simulink model "B4_quadcopter_model_discrete"  (R2021b)
settings: Solver=VariableStepAuto  StartTime=0.0  StopTime=10  FixedStep=0.002  RelTol=1e-3
values from neighbouring files (symbols this model uses):
  coef_sim_1 = tf_des_d.Denominator{1}(2)    [A11_setup_script_pprz.m]    (also in A1_setup_script.m; A6_slow_actuator.m)
  coef_sim_2 = tf_des_d.Numerator{1}(2)    [A11_setup_script_pprz.m]    (also in A1_setup_script.m; A6_slow_actuator.m)
  doublet_mag = - 0.15    (= -0.15)    [A11_setup_script_pprz.m]    (also in A1_setup_script.m)
  doublet_time = 6    [A11_setup_script_pprz.m]    (also in A1_setup_script.m)
  f_8 = 1    [A11_setup_script_pprz.m]    (also in A1_setup_script.m)
  FILT_CUTOFF = 2*pi*5    (= 31.4159265359)    [A11_setup_script_pprz.m]    (also in A1_setup_script.m)
  FILTER = 1    [A11_setup_script_pprz.m]    (also in A1_setup_script.m)
  G1 = inv(I)*G1_r    [A10_simple_plant.m]    (also in A11_setup_script_pprz.m = G1/scale; A1_setup_script.m = [G1;G1_T])
  G1_simple = inv(I)*G1_r_simple    [A1_setup_script.m]
  G2 = G2/scale    [A11_setup_script_pprz.m]    (also in A1_setup_script.m = (1/sampling_time)*inv(I)*(G2_r))
  h_plate = 0.3    [A11_setup_script_pprz.m]    (also in A1_setup_script.m = 0.16)
  I = eye(3,3)    [A10_simple_plant.m]    (also in A11_setup_script_pprz.m; A1_setup_script.m; A2_B_matrix_generation_symbolic.m = [Ixx 0 0; A3_B_matrix_generation_symbolic_cascaded.m = [Ixx 0 0)
  Iyy = 0.0008    [A11_setup_script_pprz.m]    (also in A1_setup_script.m = 0.0015)
  Izz = 0.000498    [A11_setup_script_pprz.m]    (also in A1_setup_script.m = 0.00015)
  K = 7    [A11_setup_script_pprz.m]    (also in A1_setup_script.m = 10)
  K_act = 50    [A10_simple_plant.m]    (also in A11_setup_script_pprz.m = 20; A1_setup_script.m = 20)
  K_act_outer = diag([K K K_act])    [A1_setup_script.m]
  K_d = 15    [A11_setup_script_pprz.m]    (also in A1_setup_script.m = 25)
  K_dd = K_act    (= 20)    [A11_setup_script_pprz.m]    (also in A1_setup_script.m)
  K_dyn = K    (= 10)    [A1_setup_script.m]
  K_ec = 50    [A11_setup_script_pprz.m]    (also in A1_setup_script.m = 251)
  K_ec_d = 13    [A11_setup_script_pprz.m]    (also in A1_setup_script.m = 25)
  K_ec_d_u = 1.5    [A11_setup_script_pprz.m]    (also in A1_setup_script.m = 5)
  K_ec_d_v = 1.5    [A11_setup_script_pprz.m]    (also in A1_setup_script.m = 5)
  K_ec_d_w = 1.5    [A11_setup_script_pprz.m]    (also in A1_setup_script.m = 5)
  K_ec_dd = 9    [A11_setup_script_pprz.m]    (also in A1_setup_script.m = 45)
  K_ec_i = 0    [A11_setup_script_pprz.m]    (also in A1_setup_script.m = 380)
  K_ec_u = 1.5    [A11_setup_script_pprz.m]    (also in A1_setup_script.m = 5)
  K_ec_v = 1.5    [A11_setup_script_pprz.m]    (also in A1_setup_script.m = 5)
  K_ec_w = 1.5    [A11_setup_script_pprz.m]    (also in A1_setup_script.m = 5)
  K_t = 0.0005    [A10_simple_plant.m]    (also in A11_setup_script_pprz.m = 6.557e-08; A1_setup_script.m = 6.557e-08)
  K_u = 1.0    (= 1)    [A11_setup_script_pprz.m]    (also in A1_setup_script.m = 1.5)
  K_u_d = 2.5    [A11_setup_script_pprz.m]    (also in A1_setup_script.m = 7)
  K_u_dd = K    (= 10)    [A1_setup_script.m]
  K_v = 1.0    (= 1)    [A11_setup_script_pprz.m]    (also in A1_setup_script.m = 1.5)
  K_v_d = 2.5    [A11_setup_script_pprz.m]    (also in A1_setup_script.m = 7)
  K_v_dd = K    (= 10)    [A1_setup_script.m]
  K_w = 1.0    (= 1)    [A11_setup_script_pprz.m]    (also in A1_setup_script.m = 4.5)
  K_w_d = 2.5    [A11_setup_script_pprz.m]    (also in A1_setup_script.m = 7)
  K_w_dd = K    (= 10)    [A1_setup_script.m]
  l_plate = 0.1    [A11_setup_script_pprz.m]    (also in A1_setup_script.m = 0.11)
  m = 0.4    [A10_simple_plant.m]    (also in A11_setup_script_pprz.m; A1_setup_script.m)
  NOISE = 0    [A11_setup_script_pprz.m]    (also in A1_setup_script.m)
  NOISE_ACC = 0.00005    (= 5e-05)    [A11_setup_script_pprz.m]    (also in A1_setup_script.m)
  NOISE_GYRO = 0.00005    (= 5e-05)    [A11_setup_script_pprz.m]    (also in A1_setup_script.m)
  NOISE_RPM = 200    [A11_setup_script_pprz.m]    (also in A1_setup_script.m)
  omega_act = 50    [A6_slow_actuator.m]
  omega_des = 20.00    (= 20)    [A11_setup_script_pprz.m]    (also in A1_setup_script.m; A6_slow_actuator.m = 49)
  sampling_time = 1/frequency    (= 0.002)    [A11_setup_script_pprz.m]    (also in A12_sim_multi_run.m; A1_setup_script.m; A6_slow_actuator.m)
  scale_8 = 1.6    [A11_setup_script_pprz.m]    (also in A1_setup_script.m)
  start_8 = 2    [A11_setup_script_pprz.m]    (also in A1_setup_script.m)
  start_time = 2    [A11_setup_script_pprz.m]    (also in A1_setup_script.m = 1)
  t_8 = 10    [A11_setup_script_pprz.m]    (also in A1_setup_script.m)
  w_plate = 0.3    [A11_setup_script_pprz.m]    (also in A1_setup_script.m = 0.36)
undefined symbols (not defined in the file or in its folder): DiscIntNeverNeededParam, K_ec_d_p, K_ec_d_q, K_ec_d_r, K_ec_dd_p, K_ec_dd_q, K_ec_dd_r, K_ec_i_u, K_ec_i_v, K_ec_i_w, K_ec_p, K_ec_q, K_ec_r, K_p, K_p_d, K_p_dd, K_q, K_q_d, K_q_dd, K_r, K_r_d, K_r_dd
libraries: simulink x44, cstblocks x37, dspinverses x26, dspmathops x9, dspstat3 x9, aerolibutil x9, sharedutil x3, aerolibanim x1
(part 10 of 13)

== system B4_quadcopter_model_discrete/Discrete Model/Discrete INDI Controller Cascaded w// Actuator Compensation1/INTERNAL REFERENCE MODEL ATTITUDE/body rates to euler rates ==
  p : Inport
  q : Inport  Port=2
  r : Inport  Port=3
  Demux : Demux  Outputs=3
  Matrix Multiply : Product  Multiplication=Matrix(*)
  Mux : Mux  Inputs=3
  phi_dot : Outport
  theta_dot : Outport  Port=2
  psi_dot : Outport  Port=3
  wires:
  p/1 -> Mux/1
  q/1 -> Mux/2
  r/1 -> Mux/3
  [T_discr] -> Matrix Multiply/1
  Mux/1 -> Matrix Multiply/2
  Matrix Multiply/1 -> Demux/1
  Demux/3 -> psi_dot/1
  Demux/2 -> theta_dot/1
  Demux/1 -> phi_dot/1

== system B4_quadcopter_model_discrete/Discrete Model/Discrete INDI Controller Cascaded w// Actuator Compensation1/INTERNAL REFERENCE MODEL ATTITUDE/euler rates to body rates ==
  phi_dot : Inport
  theta_dot : Inport  Port=2
  psi_dot : Inport  Port=3
  Demux : Demux  Outputs=3
  Matrix Multiply : Product  Multiplication=Matrix(*)
  Mux : Mux  Inputs=3
  p : Outport
  q : Outport  Port=2
  r : Outport  Port=3
  wires:
  phi_dot/1 -> Mux/1
  theta_dot/1 -> Mux/2
  psi_dot/1 -> Mux/3
  [R_discr] -> Matrix Multiply/1
  Mux/1 -> Matrix Multiply/2
  Matrix Multiply/1 -> Demux/1
  Demux/3 -> r/1
  Demux/2 -> q/1
  Demux/1 -> p/1

== system B4_quadcopter_model_discrete/Discrete Model/Plant and State Estimation/Butterworth Lowpass 2nd Order1/Switch Case Action Subsystem ==
  In1 : Inport
  Action Port : ActionPort  ActionPortLabel=case [ 1 ]:
  Constant5 : Constant  Value=FILT_CUTOFF  SampleTime=sampling_time
  Lowpass2 : cstblocks/Linear Parameter Varying/Discrete Varying Lowpass  N=2  w0=0  Ts=sampling_time
      settings: SourceProductBaseCode=CT
  Out1 : Outport
  wires:
  Constant5/1 -> Lowpass2/2
  In1/1 -> Lowpass2/1
  Lowpass2/1 -> Out1/1

== system B4_quadcopter_model_discrete/Discrete Model/Plant and State Estimation/Butterworth Lowpass 2nd Order1/Switch Case Action Subsystem1 ==
  In1 : Inport
  Action Port : ActionPort  ActionPortLabel=default:
  Out1 : Outport
  wires:
  In1/1 -> Out1/1

== system B4_quadcopter_model_discrete/Discrete Model/Plant and State Estimation/Butterworth Lowpass 2nd Order2/Switch Case Action Subsystem ==
  In1 : Inport
  Action Port : ActionPort  ActionPortLabel=case [ 1 ]:
  Constant5 : Constant  Value=FILT_CUTOFF  SampleTime=sampling_time
  Lowpass2 : cstblocks/Linear Parameter Varying/Discrete Varying Lowpass  N=2  w0=0  Ts=sampling_time
      settings: SourceProductBaseCode=CT
  Out1 : Outport
  wires:
  Constant5/1 -> Lowpass2/2
  In1/1 -> Lowpass2/1
  Lowpass2/1 -> Out1/1

== system B4_quadcopter_model_discrete/Discrete Model/Plant and State Estimation/Butterworth Lowpass 2nd Order2/Switch Case Action Subsystem1 ==
  In1 : Inport
  Action Port : ActionPort  ActionPortLabel=default:
  Out1 : Outport
  wires:
  In1/1 -> Out1/1

== system B4_quadcopter_model_discrete/Discrete Model/Plant and State Estimation/Butterworth Lowpass 2nd Order3/Switch Case Action Subsystem ==
  In1 : Inport
  Action Port : ActionPort  ActionPortLabel=case [ 1 ]:
  Constant5 : Constant  Value=FILT_CUTOFF  SampleTime=sampling_time
  Lowpass2 : cstblocks/Linear Parameter Varying/Discrete Varying Lowpass  N=2  w0=0  Ts=sampling_time
      settings: SourceProductBaseCode=CT
  Out1 : Outport
  wires:
  Constant5/1 -> Lowpass2/2
  In1/1 -> Lowpass2/1
  Lowpass2/1 -> Out1/1

== system B4_quadcopter_model_discrete/Discrete Model/Plant and State Estimation/Butterworth Lowpass 2nd Order3/Switch Case Action Subsystem1 ==
  In1 : Inport
  Action Port : ActionPort  ActionPortLabel=default:
  Out1 : Outport
  wires:
  In1/1 -> Out1/1

== system B4_quadcopter_model_discrete/Discrete Model/Plant and State Estimation/Butterworth Lowpass 2nd Order4/Switch Case Action Subsystem ==
  In1 : Inport
  Action Port : ActionPort  ActionPortLabel=case [ 1 ]:
  Constant5 : Constant  Value=FILT_CUTOFF  SampleTime=sampling_time
  Lowpass2 : cstblocks/Linear Parameter Varying/Discrete Varying Lowpass  N=2  w0=0  Ts=sampling_time
      settings: SourceProductBaseCode=CT
  Out1 : Outport
  wires:
  Constant5/1 -> Lowpass2/2
  In1/1 -> Lowpass2/1
  Lowpass2/1 -> Out1/1

== system B4_quadcopter_model_discrete/Discrete Model/Plant and State Estimation/Butterworth Lowpass 2nd Order4/Switch Case Action Subsystem1 ==
  In1 : Inport
  Action Port : ActionPort  ActionPortLabel=default:
  Out1 : Outport
  wires:
  In1/1 -> Out1/1

== system B4_quadcopter_model_discrete/Discrete Model/Plant and State Estimation/Butterworth Lowpass 2nd Order5/Switch Case Action Subsystem ==
  In1 : Inport
  Action Port : ActionPort  ActionPortLabel=case [ 1 ]:
  Constant5 : Constant  Value=FILT_CUTOFF  SampleTime=sampling_time
  Lowpass2 : cstblocks/Linear Parameter Varying/Discrete Varying Lowpass  N=2  w0=0  Ts=sampling_time
      settings: SourceProductBaseCode=CT
  Out1 : Outport
  wires:
  Constant5/1 -> Lowpass2/2
  In1/1 -> Lowpass2/1
  Lowpass2/1 -> Out1/1

== system B4_quadcopter_model_discrete/Discrete Model/Plant and State Estimation/Butterworth Lowpass 2nd Order5/Switch Case Action Subsystem1 ==
  In1 : Inport
  Action Port : ActionPort  ActionPortLabel=default:
  Out1 : Outport
  wires:
  In1/1 -> Out1/1

== system B4_quadcopter_model_discrete/Discrete Model/Plant and State Estimation/Plant Dynamics Continuous/Disturbance Block ==
  Step : Step  Time=2  After=60  SampleTime=0
  Sum : Sum  Inputs=|++
  Total Disturbance : Outport
  wires:
  Step/1 -> Sum/1
  Sum/1 -> Total Disturbance/1

== system B4_quadcopter_model_discrete/Discrete Model/Plant and State Estimation/Plant Dynamics Continuous/Omega_I_Omega1 ==
  pqr_body : Inport
  Inertia : Inport  Port=2
  3x3 Cross Product : sharedutil/3x3 Cross Product  aMode=aMode
      settings: SourceProductBaseCode=AE,PW,DR,MT,UV,VE
  Matrix Multiply1 : Product  Multiplication=Matrix(*)
  Final product : Outport
  wires:
  Inertia/1 -> Matrix Multiply1/1
  Matrix Multiply1/1 -> 3x3 Cross Product/2
  3x3 Cross Product/1 -> Final product/1
  pqr_body/1 -> 3x3 Cross Product/1, Matrix Multiply1/2

== system B4_quadcopter_model_discrete/Discrete Model - Complementary Filtering/Continuous Actuator Dynamics/Noise RPM/Switch Case Action Subsystem ==
  Action Port : ActionPort  ActionPortLabel=case [ 1 ]:
  RPM Noise : simulink/Sources/Band-Limited White Noise  Cov=[NOISE_RPM]  Ts=sampling_time  seed=[23341]
  Out1 : Outport
  wires:
  RPM Noise/1 -> Out1/1

== system B4_quadcopter_model_discrete/Discrete Model - Complementary Filtering/Continuous Actuator Dynamics/Noise RPM/Switch Case Action Subsystem1 ==
  Action Port : ActionPort  ActionPortLabel=default:
  Constant : Constant  Value=0  SampleTime=sampling_time
  Out1 : Outport
  wires:
  Constant/1 -> Out1/1

== system B4_quadcopter_model_discrete/Discrete Model - Complementary Filtering/Discrete INDI Controller Cascaded/INTERNAL REFERENCE MODEL ATTITUDE/body rates to euler rates ==
  p : Inport
  q : Inport  Port=2
  r : Inport  Port=3
  Demux : Demux  Outputs=3
  Matrix Multiply : Product  Multiplication=Matrix(*)
  Mux : Mux  Inputs=3
  phi_dot : Outport
  theta_dot : Outport  Port=2
  psi_dot : Outport  Port=3
  wires:
  p/1 -> Mux/1
  q/1 -> Mux/2
  r/1 -> Mux/3
  [T_discr] -> Matrix Multiply/1
  Mux/1 -> Matrix Multiply/2
  Matrix Multiply/1 -> Demux/1
  Demux/3 -> psi_dot/1
  Demux/2 -> theta_dot/1
  Demux/1 -> phi_dot/1

== system B4_quadcopter_model_discrete/Discrete Model - Complementary Filtering/Discrete INDI Controller Cascaded/INTERNAL REFERENCE MODEL ATTITUDE/euler rates to body rates ==
  phi_dot : Inport
  theta_dot : Inport  Port=2
  psi_dot : Inport  Port=3
  Demux : Demux  Outputs=3
  Matrix Multiply : Product  Multiplication=Matrix(*)
  Mux : Mux  Inputs=3
  p : Outport
  q : Outport  Port=2
  r : Outport  Port=3
  wires:
  phi_dot/1 -> Mux/1
  theta_dot/1 -> Mux/2
  psi_dot/1 -> Mux/3
  [R_discr] -> Matrix Multiply/1
  Mux/1 -> Matrix Multiply/2
  Matrix Multiply/1 -> Demux/1
  Demux/3 -> r/1
  Demux/2 -> q/1
  Demux/1 -> p/1

== system B4_quadcopter_model_discrete/Discrete Model - Complementary Filtering/Discrete INDI Controller Cascaded/Subsystem1/Doublet Block ==
  Scope : Scope
  Step : Step  Time=start_time  After=doublet_mag  SampleTime=sampling_time
  Step1 : Step  Time=start_time + doublet_time/2  After=-doublet_mag*2  SampleTime=sampling_time
  Step2 : Step  Time=start_time + doublet_time  After=0  SampleTime=sampling_time
  Sum : Sum  Inputs=|++
  Sum1 : Sum  Inputs=|++
  Out1 : Outport
  wires:
  Step/1 -> Sum/1
  Step1/1 -> Sum/2
  Sum/1 -> Sum1/1
  Sum1/1 -> Out1/1, Scope/1
  Step2/1 -> Sum1/2

== system B4_quadcopter_model_discrete/Discrete Model - Complementary Filtering/Discrete INDI Controller Cascaded w// Actuator Compensation/INTERNAL REFERENCE MODEL ATTITUDE/body rates to euler rates ==
  p : Inport
  q : Inport  Port=2
  r : Inport  Port=3
  Demux : Demux  Outputs=3
  Matrix Multiply : Product  Multiplication=Matrix(*)
  Mux : Mux  Inputs=3
  phi_dot : Outport
  theta_dot : Outport  Port=2
  psi_dot : Outport  Port=3
  wires:
  p/1 -> Mux/1
  q/1 -> Mux/2
  r/1 -> Mux/3
  [T_discr] -> Matrix Multiply/1
  Mux/1 -> Matrix Multiply/2
  Matrix Multiply/1 -> Demux/1
  Demux/3 -> psi_dot/1
  Demux/2 -> theta_dot/1
  Demux/1 -> phi_dot/1

== system B4_quadcopter_model_discrete/Discrete Model - Complementary Filtering/Discrete INDI Controller Cascaded w// Actuator Compensation/INTERNAL REFERENCE MODEL ATTITUDE/euler rates to body rates ==
  phi_dot : Inport
  theta_dot : Inport  Port=2
  psi_dot : Inport  Port=3
  Demux : Demux  Outputs=3
  Matrix Multiply : Product  Multiplication=Matrix(*)
  Mux : Mux  Inputs=3
  p : Outport
  q : Outport  Port=2
  r : Outport  Port=3
  wires:
  phi_dot/1 -> Mux/1
  theta_dot/1 -> Mux/2
  psi_dot/1 -> Mux/3
  [R_discr] -> Matrix Multiply/1
  Mux/1 -> Matrix Multiply/2
  Matrix Multiply/1 -> Demux/1
  Demux/3 -> r/1
  Demux/2 -> q/1
  Demux/1 -> p/1

== system B4_quadcopter_model_discrete/Discrete Model - Complementary Filtering/Discrete INDI Controller Cascaded w// Actuator Compensation/Subsystem/body rates to euler rates ==
  p : Inport
  q : Inport  Port=2
  r : Inport  Port=3
  Demux : Demux  Outputs=3
  Matrix Multiply : Product  Multiplication=Matrix(*)
  Mux : Mux  Inputs=3
  phi_dot : Outport
  theta_dot : Outport  Port=2
  psi_dot : Outport  Port=3
  wires:
  p/1 -> Mux/1
  q/1 -> Mux/2
  r/1 -> Mux/3
  [T_discr] -> Matrix Multiply/1
  Mux/1 -> Matrix Multiply/2
  Matrix Multiply/1 -> Demux/1
  Demux/3 -> psi_dot/1
  Demux/2 -> theta_dot/1
  Demux/1 -> phi_dot/1

== system B4_quadcopter_model_discrete/Discrete Model - Complementary Filtering/Discrete INDI Controller Cascaded w// Actuator Compensation/Subsystem/body rates to euler rates1 ==
  p : Inport
  q : Inport  Port=2
  r : Inport  Port=3
  Demux : Demux  Outputs=3
  Matrix Multiply : Product  Multiplication=Matrix(*)
  Mux : Mux  Inputs=3
  phi_dot : Outport
  theta_dot : Outport  Port=2
  psi_dot : Outport  Port=3
  wires:
  p/1 -> Mux/1
  q/1 -> Mux/2
  r/1 -> Mux/3
  [T_discr] -> Matrix Multiply/1
  Mux/1 -> Matrix Multiply/2
  Matrix Multiply/1 -> Demux/1
  Demux/3 -> psi_dot/1
  Demux/2 -> theta_dot/1
  Demux/1 -> phi_dot/1

== system B4_quadcopter_model_discrete/Discrete Model - Complementary Filtering/Discrete INDI Controller Cascaded w// Actuator Compensation/Subsystem/body rates to euler rates2 ==
  p : Inport
  q : Inport  Port=2
  r : Inport  Port=3
  Demux : Demux  Outputs=3
  Matrix Multiply : Product  Multiplication=Matrix(*)
  Mux : Mux  Inputs=3
  phi_dot : Outport
  theta_dot : Outport  Port=2
  psi_dot : Outport  Port=3
  wires:
  p/1 -> Mux/1
  q/1 -> Mux/2
  r/1 -> Mux/3
  [T_discr] -> Matrix Multiply/1
  Mux/1 -> Matrix Multiply/2
  Matrix Multiply/1 -> Demux/1
  Demux/3 -> psi_dot/1
  Demux/2 -> theta_dot/1
  Demux/1 -> phi_dot/1

== system B4_quadcopter_model_discrete/Discrete Model - Complementary Filtering/Discrete INDI Controller Cascaded w// Actuator Compensation Double/Butterworth Lowpass 2nd Order3/Switch Case Action Subsystem ==
  In1 : Inport
  Action Port : ActionPort
  Constant5 : Constant  Value=FILT_CUTOFF  SampleTime=sampling_time
  Lowpass2 : cstblocks/Linear Parameter Varying/Discrete Varying Lowpass  N=2  w0=0  Ts=sampling_time
      settings: SourceProductBaseCode=CT
  Out1 : Outport
  wires:
  Constant5/1 -> Lowpass2/2
  In1/1 -> Lowpass2/1
  Lowpass2/1 -> Out1/1

== system B4_quadcopter_model_discrete/Discrete Model - Complementary Filtering/Discrete INDI Controller Cascaded w// Actuator Compensation Double/Butterworth Lowpass 2nd Order3/Switch Case Action Subsystem1 ==
  In1 : Inport
  Action Port : ActionPort
  Out1 : Outport
  wires:
  In1/1 -> Out1/1

== system B4_quadcopter_model_discrete/Discrete Model - Complementary Filtering/Discrete INDI Controller Cascaded w// Actuator Compensation Double/INTERNAL REFERENCE MODEL ATTITUDE/body rates to euler rates ==
  p : Inport
  q : Inport  Port=2
  r : Inport  Port=3
  Demux : Demux  Outputs=3
  Matrix Multiply : Product  Multiplication=Matrix(*)
  Mux : Mux  Inputs=3
  phi_dot : Outport
  theta_dot : Outport  Port=2
  psi_dot : Outport  Port=3
  wires:
  p/1 -> Mux/1
  q/1 -> Mux/2
  r/1 -> Mux/3
  [T_discr] -> Matrix Multiply/1
  Mux/1 -> Matrix Multiply/2
  Matrix Multiply/1 -> Demux/1
  Demux/3 -> psi_dot/1
  Demux/2 -> theta_dot/1
  Demux/1 -> phi_dot/1

== system B4_quadcopter_model_discrete/Discrete Model - Complementary Filtering/Discrete INDI Controller Cascaded w// Actuator Compensation Double/INTERNAL REFERENCE MODEL ATTITUDE/euler rates to body rates ==
  phi_dot : Inport
  theta_dot : Inport  Port=2
  psi_dot : Inport  Port=3
  Demux : Demux  Outputs=3
  Matrix Multiply : Product  Multiplication=Matrix(*)
  Mux : Mux  Inputs=3
  p : Outport
  q : Outport  Port=2
  r : Outport  Port=3
  wires:
  phi_dot/1 -> Mux/1
  theta_dot/1 -> Mux/2
  psi_dot/1 -> Mux/3
  [R_discr] -> Matrix Multiply/1
  Mux/1 -> Matrix Multiply/2
  Matrix Multiply/1 -> Demux/1
  Demux/3 -> r/1
  Demux/2 -> q/1
  Demux/1 -> p/1

== system B4_quadcopter_model_discrete/Discrete Model - Complementary Filtering/Discrete INDI Controller Cascaded w// Actuator Compensation Double/Pitch Jerk Compensation/Butterworth Lowpass 2nd Order2 ==
  state estimate : Inport
  Constant5 : Constant  Value=FILT_CUTOFF  SampleTime=sampling_time
  Lowpass2 : cstblocks/Linear Parameter Varying/Discrete Varying Lowpass  N=2  w0=0  Ts=sampling_time
      settings: SourceProductBaseCode=CT
  Out : Outport
  wires:
  Constant5/1 -> Lowpass2/2
  Lowpass2/1 -> Out/1
  state estimate/1 -> Lowpass2/1

== system B4_quadcopter_model_discrete/Discrete Model - Complementary Filtering/Discrete INDI Controller Cascaded w// Actuator Compensation Double/Pitch Jerk Compensation/Model Based State Estimate ==
  Mux : Mux  Inputs=12
  state estimate : Outport
  wires:
  [Az] -> Mux/9
  [Vy] -> Mux/2
  [q] -> Mux/11
  [phi] -> Mux/4
  [Ay] -> Mux/8
  [p] -> Mux/10
  [psi] -> Mux/6
  [Ax] -> Mux/7
  [r] -> Mux/12
  [Vx] -> Mux/1
  [theta] -> Mux/5
  [Vz] -> Mux/3
  Mux/1 -> state estimate/1  "plant based"

== system B4_quadcopter_model_discrete/Discrete Model - Complementary Filtering/Discrete INDI Controller Cascaded w// Actuator Compensation Double/Pitch Jerk Compensation/State Filtered ==
  Mux : Mux  Inputs=12
  state filtered : Outport
  wires:
  [Az_f] -> Mux/9
  [Vy_f] -> Mux/2
  [q_f] -> Mux/11
  [phi_f] -> Mux/4
  [Ay_f] -> Mux/8
  [p_f] -> Mux/10
  [psi_f] -> Mux/6
  [Ax_f] -> Mux/7
  [r_f] -> Mux/12
  [Vx_f] -> Mux/1
  [theta_f] -> Mux/5
  [Vz_f] -> Mux/3
  Mux/1 -> state filtered/1  "plant based"

== system B4_quadcopter_model_discrete/Discrete Model - Complementary Filtering/Discrete INDI Controller Cascaded w// Actuator Compensation Double/Pitch Jerk Compensation CopyPaste/Aero Package Easy ==
  Constant : Constant  Value=0
  Constant2 : Constant  Value=w_plate
  Constant3 : Constant  Value=h_plate
  Constant5 : Constant  Value=l_plate
  Mux : Mux  Inputs=3
  Mux1 : Mux  Inputs=3
  Terminator : Terminator
  Terminator1 : Terminator
  drag plate My : MATLAB Function  TreatAsAtomicUnit=on
  Aero Moment : Outport
  Aero Force : Outport  Port=2
  wires:
  Mux/1 -> Aero Moment/1  "aero_moment"
  Constant/1 -> Mux1/2, Mux/3, Mux/1
  drag plate My/1(My_dp) -> Mux/2  "My_dp"
  drag plate My/2(Fx_earth) -> Mux1/1  "Fx_aero_earth"
  Constant2/1 -> drag plate My/1(w_plate)
  Constant3/1 -> drag plate My/2(h_plate)
  Constant5/1 -> drag plate My/3(l_plate)
  [theta_cont] -> drag plate My/4(theta)
  Mux1/1 -> Aero Force/1  "aero_force"
  drag plate My/3(Fz_earth) -> Mux1/3  "Fz_aero_earth"
  drag plate My/4(Cl) -> Terminator/1  "Cl"
  drag plate My/5(Cd) -> Terminator1/1  "Cd"
  [u_cont] -> drag plate My/5(u)
  [w_cont] -> drag plate My/6(w)

== system B4_quadcopter_model_discrete/Discrete Model - Complementary Filtering/Discrete INDI Controller Cascaded w// Actuator Compensation Double/Pitch Jerk Compensation1/body rates to euler rates ==
  p : Inport
  q : Inport  Port=2
  r : Inport  Port=3
  Demux : Demux  Outputs=3
  Matrix Multiply : Product  Multiplication=Matrix(*)
  Mux : Mux  Inputs=3
  phi_dot : Outport
  theta_dot : Outport  Port=2
  psi_dot : Outport  Port=3
  wires:
  p/1 -> Mux/1
  q/1 -> Mux/2
  r/1 -> Mux/3
  [T_discr] -> Matrix Multiply/1
  Mux/1 -> Matrix Multiply/2
  Matrix Multiply/1 -> Demux/1
  Demux/3 -> psi_dot/1
  Demux/2 -> theta_dot/1
  Demux/1 -> phi_dot/1

== system B4_quadcopter_model_discrete/Discrete Model - Complementary Filtering/Plant and State Estimation/Angular Velocity Model/Drag Plate Aerodynamics ==
  Constant : Constant  Value=0
  Constant2 : Constant  Value=w_plate
  Constant3 : Constant  Value=h_plate
  Constant5 : Constant  Value=l_plate
  Mux : Mux  Inputs=3
  Mux1 : Mux  Inputs=3
  Scope : Scope  NumInputPorts=2
  drag plate My : MATLAB Function  TreatAsAtomicUnit=on
  Aero Moment : Outport
  Aero Force : Outport  Port=2
  wires:
  drag plate My/2(Fx_earth) -> Mux1/1  "Fx_aero_earth"
  Constant/1 -> Mux/2, Mux/1
  [Vx_cont] -> drag plate My/5(Vx)
  drag plate My/3(Fy_earth) -> Mux1/2  "Fy_aero_earth"
  Constant5/1 -> drag plate My/3(l_plate)
  Mux1/1 -> Aero Force/1  "aero_force"
  [theta_cont] -> drag plate My/4(theta)
  [q_cont] -> drag plate My/8(q)
  drag plate My/5(D_plate_vel) -> Scope/1
  [Vy_cont] -> drag plate My/6(Vy)
  drag plate My/4(Fz_earth) -> Mux1/3  "Fz_aero_earth"
  [psi_cont] -> drag plate My/7(heading)
  Mux/1 -> Aero Moment/1  "aero_moment"
  Constant2/1 -> drag plate My/1(w_plate)
  Constant3/1 -> drag plate My/2(h_plate)
  drag plate My/6(D_plate_rot) -> Scope/2
  drag plate My/1(Mz_dp) -> Mux/3  "Mz_dp"

== system B4_quadcopter_model_discrete/Discrete Model - Complementary Filtering/Plant and State Estimation/Complementary Filter/Butterworth Lowpass 2nd Order1 ==
  In : Inport
  Constant : Constant  Value=FILTER  SampleTime=sampling_time
  Merge : Merge
  Switch Case : SwitchCase
  Switch Case Action Subsystem : Subsystem  TreatAsAtomicUnit=on
  Switch Case Action Subsystem1 : Subsystem  TreatAsAtomicUnit=on
  Out : Outport
  wires:
  Merge/1 -> Out/1
  Switch Case Action Subsystem/1(Out1) -> Merge/1
  Constant/1 -> Switch Case/1
  Switch Case Action Subsystem1/1(Out1) -> Merge/2
  Switch Case/2 -> Switch Case Action Subsystem1/Action
  In/1 -> Switch Case Action Subsystem/1(In1), Switch Case Action Subsystem1/1(In1)
  Switch Case/1 -> Switch Case Action Subsystem/Action

== system B4_quadcopter_model_discrete/Discrete Model - Complementary Filtering/Plant and State Estimation/Complementary Filter/Butterworth Lowpass 2nd Order2 ==
  In : Inport
  Constant : Constant  Value=FILTER  SampleTime=sampling_time
  Merge : Merge
  Switch Case : SwitchCase
  Switch Case Action Subsystem : Subsystem  TreatAsAtomicUnit=on
  Switch Case Action Subsystem1 : Subsystem  TreatAsAtomicUnit=on
  Out : Outport
  wires:
  Merge/1 -> Out/1
  Switch Case Action Subsystem/1(Out1) -> Merge/1
  Constant/1 -> Switch Case/1
  Switch Case Action Subsystem1/1(Out1) -> Merge/2
  Switch Case/2 -> Switch Case Action Subsystem1/Action
  In/1 -> Switch Case Action Subsystem/1(In1), Switch Case Action Subsystem1/1(In1)
  Switch Case/1 -> Switch Case Action Subsystem/Action

== system B4_quadcopter_model_discrete/Discrete Model - Complementary Filtering/Plant and State Estimation/Complementary Filter1/Butterworth Lowpass 2nd Order1 ==
  In : Inport
  Constant : Constant  Value=FILTER  SampleTime=sampling_time
  Merge : Merge
  Switch Case : SwitchCase
  Switch Case Action Subsystem : Subsystem  TreatAsAtomicUnit=on
  Switch Case Action Subsystem1 : Subsystem  TreatAsAtomicUnit=on
  Out : Outport
  wires:
  Merge/1 -> Out/1
  Switch Case Action Subsystem/1(Out1) -> Merge/1
  Constant/1 -> Switch Case/1
  Switch Case Action Subsystem1/1(Out1) -> Merge/2
  Switch Case/2 -> Switch Case Action Subsystem1/Action
  In/1 -> Switch Case Action Subsystem/1(In1), Switch Case Action Subsystem1/1(In1)
  Switch Case/1 -> Switch Case Action Subsystem/Action

== system B4_quadcopter_model_discrete/Discrete Model - Complementary Filtering/Plant and State Estimation/Complementary Filter1/Butterworth Lowpass 2nd Order2 ==
  In : Inport
  Constant : Constant  Value=FILTER  SampleTime=sampling_time
  Merge : Merge
  Switch Case : SwitchCase
  Switch Case Action Subsystem : Subsystem  TreatAsAtomicUnit=on
  Switch Case Action Subsystem1 : Subsystem  TreatAsAtomicUnit=on
  Out : Outport
  wires:
  Merge/1 -> Out/1
  Switch Case Action Subsystem/1(Out1) -> Merge/1
  Constant/1 -> Switch Case/1
  Switch Case Action Subsystem1/1(Out1) -> Merge/2
  Switch Case/2 -> Switch Case Action Subsystem1/Action
  In/1 -> Switch Case Action Subsystem/1(In1), Switch Case Action Subsystem1/1(In1)
  Switch Case/1 -> Switch Case Action Subsystem/Action

== system B4_quadcopter_model_discrete/Discrete Model - Complementary Filtering/Plant and State Estimation/Noise Acc/Switch Case Action Subsystem ==
  Action Port : ActionPort  ActionPortLabel=case [ 1 ]:
  Acc Noise : simulink/Sources/Band-Limited White Noise  Cov=[NOISE_ACC]  Ts=sampling_time  seed=[23341]
  Out1 : Outport
  wires:
  Acc Noise/1 -> Out1/1

== system B4_quadcopter_model_discrete/Discrete Model - Complementary Filtering/Plant and State Estimation/Noise Acc/Switch Case Action Subsystem1 ==
  Action Port : ActionPort  ActionPortLabel=default:
  Constant : Constant  Value=0  SampleTime=sampling_time
  Out1 : Outport
  wires:
  Constant/1 -> Out1/1

== system B4_quadcopter_model_discrete/Discrete Model - Complementary Filtering/Plant and State Estimation/Noise Gyro/Switch Case Action Subsystem ==
  Action Port : ActionPort  ActionPortLabel=case [ 1 ]:
  Gyro Noise : simulink/Sources/Band-Limited White Noise  Cov=[NOISE_GYRO]  Ts=sampling_time  seed=[23341]
  Out1 : Outport
  wires:
  Gyro Noise/1 -> Out1/1

== system B4_quadcopter_model_discrete/Discrete Model - Complementary Filtering/Plant and State Estimation/Noise Gyro/Switch Case Action Subsystem1 ==
  Action Port : ActionPort  ActionPortLabel=default:
  Constant : Constant  Value=0  SampleTime=sampling_time
  Out1 : Outport
  wires:
  Constant/1 -> Out1/1

== system B4_quadcopter_model_discrete/Discrete Model - Complementary Filtering/Plant and State Estimation/Plant Dynamics Continuous/Disturbance Block ==
  Step : Step  Time=2  After=60  SampleTime=0
  Sum : Sum  Inputs=|++
  Total Disturbance : Outport
  wires:
  Step/1 -> Sum/1
  Sum/1 -> Total Disturbance/1

== system B4_quadcopter_model_discrete/Discrete Model - Complementary Filtering/Plant and State Estimation/Plant Dynamics Continuous/Omega_I_Omega1 ==
  pqr_body : Inport
  Inertia : Inport  Port=2
  3x3 Cross Product : sharedutil/3x3 Cross Product  aMode=aMode
      settings: SourceProductBaseCode=AE,PW,DR,MT,UV,VE
  Matrix Multiply1 : Product  Multiplication=Matrix(*)
  Final product : Outport
  wires:
  Inertia/1 -> Matrix Multiply1/1
  Matrix Multiply1/1 -> 3x3 Cross Product/2
  3x3 Cross Product/1 -> Final product/1
  pqr_body/1 -> 3x3 Cross Product/1, Matrix Multiply1/2

== system B4_quadcopter_model_discrete/Discrete Model - Doublet/Continuous Actuator Dynamics/Butterworth Lowpass 2nd Order1/Switch Case Action Subsystem ==
  In1 : Inport
  Action Port : ActionPort  ActionPortLabel=case [ 1 ]:
  Constant5 : Constant  Value=FILT_CUTOFF  SampleTime=sampling_time
  Lowpass2 : cstblocks/Linear Parameter Varying/Discrete Varying Lowpass  N=2  w0=0  Ts=sampling_time
      settings: SourceProductBaseCode=CT
  Out1 : Outport
  wires:
  Constant5/1 -> Lowpass2/2
  In1/1 -> Lowpass2/1
  Lowpass2/1 -> Out1/1

== system B4_quadcopter_model_discrete/Discrete Model - Doublet/Continuous Actuator Dynamics/Butterworth Lowpass 2nd Order1/Switch Case Action Subsystem1 ==
  In1 : Inport
  Action Port : ActionPort  ActionPortLabel=default:
  Out1 : Outport
  wires:
  In1/1 -> Out1/1

== system B4_quadcopter_model_discrete/Discrete Model - Doublet/Discrete INDI Controller Cascaded/INTERNAL REFERENCE MODEL ATTITUDE/body rates to euler rates ==
  p : Inport
  q : Inport  Port=2
  r : Inport  Port=3
  Demux : Demux  Outputs=3
  Matrix Multiply : Product  Multiplication=Matrix(*)
  Mux : Mux  Inputs=3
  phi_dot : Outport
  theta_dot : Outport  Port=2
  psi_dot : Outport  Port=3
  wires:
  p/1 -> Mux/1
  q/1 -> Mux/2
  r/1 -> Mux/3
  [T_discr] -> Matrix Multiply/1
  Mux/1 -> Matrix Multiply/2
  Matrix Multiply/1 -> Demux/1
  Demux/3 -> psi_dot/1
  Demux/2 -> theta_dot/1
  Demux/1 -> phi_dot/1

== system B4_quadcopter_model_discrete/Discrete Model - Doublet/Discrete INDI Controller Cascaded/INTERNAL REFERENCE MODEL ATTITUDE/euler rates to body rates ==
  phi_dot : Inport
  theta_dot : Inport  Port=2
  psi_dot : Inport  Port=3
  Demux : Demux  Outputs=3
  Matrix Multiply : Product  Multiplication=Matrix(*)
  Mux : Mux  Inputs=3
  p : Outport
  q : Outport  Port=2
  r : Outport  Port=3
  wires:
  phi_dot/1 -> Mux/1
  theta_dot/1 -> Mux/2
  psi_dot/1 -> Mux/3
  [R_discr] -> Matrix Multiply/1
  Mux/1 -> Matrix Multiply/2
  Matrix Multiply/1 -> Demux/1
  Demux/3 -> r/1
  Demux/2 -> q/1
  Demux/1 -> p/1

== system B4_quadcopter_model_discrete/Discrete Model - Doublet/Discrete INDI Controller Cascaded/Subsystem/Doublet Block ==
  Scope : Scope
  Step : Step  Time=start_time  After=doublet_mag  SampleTime=sampling_time
  Step1 : Step  Time=start_time + doublet_time/2  After=-doublet_mag*2  SampleTime=sampling_time
  Step2 : Step  Time=start_time + doublet_time  After=0  SampleTime=sampling_time
  Sum : Sum  Inputs=|++
  Sum1 : Sum  Inputs=|++
  Out1 : Outport
  wires:
  Step/1 -> Sum/1
  Step1/1 -> Sum/2
  Sum/1 -> Sum1/1
  Sum1/1 -> Out1/1, Scope/1
  Step2/1 -> Sum1/2

== system B4_quadcopter_model_discrete/Discrete Model - Doublet/Discrete INDI Controller Cascaded w// Actuator Compensation/INTERNAL REFERENCE MODEL ATTITUDE/body rates to euler rates ==
  p : Inport
  q : Inport  Port=2
  r : Inport  Port=3
  Demux : Demux  Outputs=3
  Matrix Multiply : Product  Multiplication=Matrix(*)
  Mux : Mux  Inputs=3
  phi_dot : Outport
  theta_dot : Outport  Port=2
  psi_dot : Outport  Port=3
  wires:
  p/1 -> Mux/1
  q/1 -> Mux/2
  r/1 -> Mux/3
  [T_discr] -> Matrix Multiply/1
  Mux/1 -> Matrix Multiply/2
  Matrix Multiply/1 -> Demux/1
  Demux/3 -> psi_dot/1
  Demux/2 -> theta_dot/1
  Demux/1 -> phi_dot/1

== system B4_quadcopter_model_discrete/Discrete Model - Doublet/Discrete INDI Controller Cascaded w// Actuator Compensation/INTERNAL REFERENCE MODEL ATTITUDE/euler rates to body rates ==
  phi_dot : Inport
  theta_dot : Inport  Port=2
  psi_dot : Inport  Port=3
  Demux : Demux  Outputs=3
  Matrix Multiply : Product  Multiplication=Matrix(*)
  Mux : Mux  Inputs=3
  p : Outport
  q : Outport  Port=2
  r : Outport  Port=3
  wires:
  phi_dot/1 -> Mux/1
  theta_dot/1 -> Mux/2
  psi_dot/1 -> Mux/3
  [R_discr] -> Matrix Multiply/1
  Mux/1 -> Matrix Multiply/2
  Matrix Multiply/1 -> Demux/1
  Demux/3 -> r/1
  Demux/2 -> q/1
  Demux/1 -> p/1

== system B4_quadcopter_model_discrete/Discrete Model - Doublet/Discrete INDI Controller Cascaded w// Actuator Compensation/Subsystem/Doublet Block ==
  Scope : Scope
  Step : Step  Time=start_time  After=doublet_mag  SampleTime=sampling_time
  Step1 : Step  Time=start_time + doublet_time/2  After=-doublet_mag*2  SampleTime=sampling_time
  Step2 : Step  Time=start_time + doublet_time  After=0  SampleTime=sampling_time
  Sum : Sum  Inputs=|++
  Sum1 : Sum  Inputs=|++
  Out1 : Outport
  wires:
  Step/1 -> Sum/1
  Step1/1 -> Sum/2
  Sum/1 -> Sum1/1
  Sum1/1 -> Out1/1, Scope/1
  Step2/1 -> Sum1/2

== system B4_quadcopter_model_discrete/Discrete Model - Doublet/Discrete INDI Controller Cascaded w// Actuator Compensation Double/Butterworth Lowpass 2nd Order3/Switch Case Action Subsystem ==
  In1 : Inport
  Action Port : ActionPort
  Constant5 : Constant  Value=FILT_CUTOFF  SampleTime=sampling_time
  Lowpass2 : cstblocks/Linear Parameter Varying/Discrete Varying Lowpass  N=2  w0=0  Ts=sampling_time
      settings: SourceProductBaseCode=CT
  Out1 : Outport
  wires:
  Constant5/1 -> Lowpass2/2
  In1/1 -> Lowpass2/1
  Lowpass2/1 -> Out1/1

== system B4_quadcopter_model_discrete/Discrete Model - Doublet/Discrete INDI Controller Cascaded w// Actuator Compensation Double/Butterworth Lowpass 2nd Order3/Switch Case Action Subsystem1 ==
  In1 : Inport
  Action Port : ActionPort
  Out1 : Outport
  wires:
  In1/1 -> Out1/1

== system B4_quadcopter_model_discrete/Discrete Model - Doublet/Discrete INDI Controller Cascaded w// Actuator Compensation Double/INTERNAL REFERENCE MODEL ATTITUDE/body rates to euler rates ==
  p : Inport
  q : Inport  Port=2
  r : Inport  Port=3
  Demux : Demux  Outputs=3
  Matrix Multiply : Product  Multiplication=Matrix(*)
  Mux : Mux  Inputs=3
  phi_dot : Outport
  theta_dot : Outport  Port=2
  psi_dot : Outport  Port=3
  wires:
  p/1 -> Mux/1
  q/1 -> Mux/2
  r/1 -> Mux/3
  [T_discr] -> Matrix Multiply/1
  Mux/1 -> Matrix Multiply/2
  Matrix Multiply/1 -> Demux/1
  Demux/3 -> psi_dot/1
  Demux/2 -> theta_dot/1
  Demux/1 -> phi_dot/1

== system B4_quadcopter_model_discrete/Discrete Model - Doublet/Discrete INDI Controller Cascaded w// Actuator Compensation Double/INTERNAL REFERENCE MODEL ATTITUDE/euler rates to body rates ==
  phi_dot : Inport
  theta_dot : Inport  Port=2
  psi_dot : Inport  Port=3
  Demux : Demux  Outputs=3
  Matrix Multiply : Product  Multiplication=Matrix(*)
  Mux : Mux  Inputs=3
  p : Outport
  q : Outport  Port=2
  r : Outport  Port=3
  wires:
  phi_dot/1 -> Mux/1
  theta_dot/1 -> Mux/2
  psi_dot/1 -> Mux/3
  [R_discr] -> Matrix Multiply/1
  Mux/1 -> Matrix Multiply/2
  Matrix Multiply/1 -> Demux/1
  Demux/3 -> r/1
  Demux/2 -> q/1
  Demux/1 -> p/1

== system B4_quadcopter_model_discrete/Discrete Model - Doublet/Discrete INDI Controller Cascaded w// Actuator Compensation Double/Pitch Jerk Compensation/Butterworth Lowpass 2nd Order2 ==
  state estimate : Inport
  Constant5 : Constant  Value=FILT_CUTOFF  SampleTime=sampling_time
  Lowpass2 : cstblocks/Linear Parameter Varying/Discrete Varying Lowpass  N=2  w0=0  Ts=sampling_time
      settings: SourceProductBaseCode=CT
  Out : Outport
  wires:
  Constant5/1 -> Lowpass2/2
  Lowpass2/1 -> Out/1
  state estimate/1 -> Lowpass2/1

== system B4_quadcopter_model_discrete/Discrete Model - Doublet/Discrete INDI Controller Cascaded w// Actuator Compensation Double/Pitch Jerk Compensation/Model Based State Estimate ==
  Mux : Mux  Inputs=12
  state estimate : Outport
  wires:
  [Az] -> Mux/9
  [Vy] -> Mux/2
  [q] -> Mux/11
  [phi] -> Mux/4
  [Ay] -> Mux/8
  [p] -> Mux/10
  [psi] -> Mux/6
  [Ax] -> Mux/7
  [r] -> Mux/12
  [Vx] -> Mux/1
  [theta] -> Mux/5
  [Vz] -> Mux/3
  Mux/1 -> state estimate/1  "plant based"

== system B4_quadcopter_model_discrete/Discrete Model - Doublet/Discrete INDI Controller Cascaded w// Actuator Compensation Double/Pitch Jerk Compensation/State Filtered ==
  Mux : Mux  Inputs=12
  state filtered : Outport
  wires:
  [Az_f] -> Mux/9
  [Vy_f] -> Mux/2
  [q_f] -> Mux/11
  [phi_f] -> Mux/4
  [Ay_f] -> Mux/8
  [p_f] -> Mux/10
  [psi_f] -> Mux/6
  [Ax_f] -> Mux/7
  [r_f] -> Mux/12
  [Vx_f] -> Mux/1
  [theta_f] -> Mux/5
  [Vz_f] -> Mux/3
  Mux/1 -> state filtered/1  "plant based"

== system B4_quadcopter_model_discrete/Discrete Model - Doublet/Discrete INDI Controller Cascaded w// Actuator Compensation Double/Pitch Jerk Compensation CopyPaste/Aero Package Easy ==
  Constant : Constant  Value=0
  Constant2 : Constant  Value=w_plate
  Constant3 : Constant  Value=h_plate
  Constant5 : Constant  Value=l_plate
  Mux : Mux  Inputs=3
  Mux1 : Mux  Inputs=3
  Terminator : Terminator
  Terminator1 : Terminator
  drag plate My : MATLAB Function  TreatAsAtomicUnit=on
  Aero Moment : Outport
  Aero Force : Outport  Port=2
  wires:
  Mux/1 -> Aero Moment/1  "aero_moment"
  Constant/1 -> Mux1/2, Mux/3, Mux/1
  drag plate My/1(My_dp) -> Mux/2  "My_dp"
  drag plate My/2(Fx_earth) -> Mux1/1  "Fx_aero_earth"
  Constant2/1 -> drag plate My/1(w_plate)
  Constant3/1 -> drag plate My/2(h_plate)
  Constant5/1 -> drag plate My/3(l_plate)
  [theta_cont] -> drag plate My/4(theta)
  Mux1/1 -> Aero Force/1  "aero_force"
  drag plate My/3(Fz_earth) -> Mux1/3  "Fz_aero_earth"
  drag plate My/4(Cl) -> Terminator/1  "Cl"
  drag plate My/5(Cd) -> Terminator1/1  "Cd"
  [u_cont] -> drag plate My/5(u)
  [w_cont] -> drag plate My/6(w)

== system B4_quadcopter_model_discrete/Discrete Model - Doublet/Discrete INDI Controller Cascaded w// Actuator Compensation Double/Pitch Jerk Compensation1/body rates to euler rates ==
  p : Inport
  q : Inport  Port=2
  r : Inport  Port=3
  Demux : Demux  Outputs=3
  Matrix Multiply : Product  Multiplication=Matrix(*)
  Mux : Mux  Inputs=3
  phi_dot : Outport
  theta_dot : Outport  Port=2
  psi_dot : Outport  Port=3
  wires:
  p/1 -> Mux/1
  q/1 -> Mux/2
  r/1 -> Mux/3
  [T_discr] -> Matrix Multiply/1
  Mux/1 -> Matrix Multiply/2
  Matrix Multiply/1 -> Demux/1
  Demux/3 -> psi_dot/1
  Demux/2 -> theta_dot/1
  Demux/1 -> phi_dot/1

== system B4_quadcopter_model_discrete/Discrete Model - Doublet/Plant and State Estimation/Butterworth Lowpass 2nd Order1/Switch Case Action Subsystem ==
  In1 : Inport
  Action Port : ActionPort  ActionPortLabel=case [ 1 ]:
  Constant5 : Constant  Value=FILT_CUTOFF  SampleTime=sampling_time
  Lowpass2 : cstblocks/Linear Parameter Varying/Discrete Varying Lowpass  N=2  w0=0  Ts=sampling_time
      settings: SourceProductBaseCode=CT
  Out1 : Outport
  wires:
  Constant5/1 -> Lowpass2/2
  In1/1 -> Lowpass2/1
  Lowpass2/1 -> Out1/1

== system B4_quadcopter_model_discrete/Discrete Model - Doublet/Plant and State Estimation/Butterworth Lowpass 2nd Order1/Switch Case Action Subsystem1 ==
  In1 : Inport
  Action Port : ActionPort  ActionPortLabel=default:
  Out1 : Outport
  wires:
  In1/1 -> Out1/1

== system B4_quadcopter_model_discrete/Discrete Model - Doublet/Plant and State Estimation/Butterworth Lowpass 2nd Order2/Switch Case Action Subsystem ==
  In1 : Inport
  Action Port : ActionPort  ActionPortLabel=case [ 1 ]:
  Constant5 : Constant  Value=FILT_CUTOFF  SampleTime=sampling_time
  Lowpass2 : cstblocks/Linear Parameter Varying/Discrete Varying Lowpass  N=2  w0=0  Ts=sampling_time
      settings: SourceProductBaseCode=CT
  Out1 : Outport
  wires:
  Constant5/1 -> Lowpass2/2
  In1/1 -> Lowpass2/1
  Lowpass2/1 -> Out1/1

== system B4_quadcopter_model_discrete/Discrete Model - Doublet/Plant and State Estimation/Butterworth Lowpass 2nd Order2/Switch Case Action Subsystem1 ==
  In1 : Inport
  Action Port : ActionPort  ActionPortLabel=default:
  Out1 : Outport
  wires:
  In1/1 -> Out1/1

== system B4_quadcopter_model_discrete/Discrete Model - Doublet/Plant and State Estimation/Butterworth Lowpass 2nd Order3/Switch Case Action Subsystem ==
  In1 : Inport
  Action Port : ActionPort  ActionPortLabel=case [ 1 ]:
  Constant5 : Constant  Value=FILT_CUTOFF  SampleTime=sampling_time
  Lowpass2 : cstblocks/Linear Parameter Varying/Discrete Varying Lowpass  N=2  w0=0  Ts=sampling_time
      settings: SourceProductBaseCode=CT
  Out1 : Outport
  wires:
  Constant5/1 -> Lowpass2/2
  In1/1 -> Lowpass2/1
  Lowpass2/1 -> Out1/1

== system B4_quadcopter_model_discrete/Discrete Model - Doublet/Plant and State Estimation/Butterworth Lowpass 2nd Order3/Switch Case Action Subsystem1 ==
  In1 : Inport
  Action Port : ActionPort  ActionPortLabel=default:
  Out1 : Outport
  wires:
  In1/1 -> Out1/1

== system B4_quadcopter_model_discrete/Discrete Model - Doublet/Plant and State Estimation/Butterworth Lowpass 2nd Order4/Switch Case Action Subsystem ==
  In1 : Inport
  Action Port : ActionPort  ActionPortLabel=case [ 1 ]:
  Constant5 : Constant  Value=FILT_CUTOFF  SampleTime=sampling_time
  Lowpass2 : cstblocks/Linear Parameter Varying/Discrete Varying Lowpass  N=2  w0=0  Ts=sampling_time
      settings: SourceProductBaseCode=CT
  Out1 : Outport
  wires:
  Constant5/1 -> Lowpass2/2
  In1/1 -> Lowpass2/1
  Lowpass2/1 -> Out1/1

== system B4_quadcopter_model_discrete/Discrete Model - Doublet/Plant and State Estimation/Butterworth Lowpass 2nd Order4/Switch Case Action Subsystem1 ==
  In1 : Inport
  Action Port : ActionPort  ActionPortLabel=default:
  Out1 : Outport
  wires:
  In1/1 -> Out1/1

== system B4_quadcopter_model_discrete/Discrete Model - Doublet/Plant and State Estimation/Plant Dynamics Continuous/Disturbance Block ==
  Step : Step  Time=2  After=60  SampleTime=0
  Sum : Sum  Inputs=|++
  Total Disturbance : Outport
  wires:
  Step/1 -> Sum/1
  Sum/1 -> Total Disturbance/1

== system B4_quadcopter_model_discrete/Discrete Model - Doublet/Plant and State Estimation/Plant Dynamics Continuous/Omega_I_Omega1 ==
  pqr_body : Inport
  Inertia : Inport  Port=2
  3x3 Cross Product : sharedutil/3x3 Cross Product  aMode=aMode
      settings: SourceProductBaseCode=AE,PW,DR,MT,UV,VE
  Matrix Multiply1 : Product  Multiplication=Matrix(*)
  Final product : Outport
  wires:
  Inertia/1 -> Matrix Multiply1/1
  Matrix Multiply1/1 -> 3x3 Cross Product/2
  3x3 Cross Product/1 -> Final product/1
  pqr_body/1 -> 3x3 Cross Product/1, Matrix Multiply1/2

== system B4_quadcopter_model_discrete/Discrete Model - Inner Loop Only/Continuous Actuator Dynamics/Butterworth Lowpass 2nd Order1/Switch Case Action Subsystem ==
  In1 : Inport
  Action Port : ActionPort  ActionPortLabel=case [ 1 ]:
  Constant5 : Constant  Value=FILT_CUTOFF  SampleTime=sampling_time
  Lowpass2 : cstblocks/Linear Parameter Varying/Discrete Varying Lowpass  N=2  w0=0  Ts=sampling_time
      settings: SourceProductBaseCode=CT
  Out1 : Outport
  wires:
  Constant5/1 -> Lowpass2/2
  In1/1 -> Lowpass2/1
  Lowpass2/1 -> Out1/1

== system B4_quadcopter_model_discrete/Discrete Model - Inner Loop Only/Continuous Actuator Dynamics/Butterworth Lowpass 2nd Order1/Switch Case Action Subsystem1 ==
  In1 : Inport
  Action Port : ActionPort  ActionPortLabel=default:
  Out1 : Outport
  wires:
  In1/1 -> Out1/1

== system B4_quadcopter_model_discrete/Discrete Model - Inner Loop Only/Discrete INDI Controller Cascaded/INTERNAL REFERENCE MODEL ATTITUDE/body rates to euler rates ==
  p : Inport
  q : Inport  Port=2
  r : Inport  Port=3
  Demux : Demux  Outputs=3
  Matrix Multiply : Product  Multiplication=Matrix(*)
  Mux : Mux  Inputs=3
  phi_dot : Outport
  theta_dot : Outport  Port=2
  psi_dot : Outport  Port=3
  wires:
  p/1 -> Mux/1
  q/1 -> Mux/2
  r/1 -> Mux/3
  [T_discr] -> Matrix Multiply/1
  Mux/1 -> Matrix Multiply/2
  Matrix Multiply/1 -> Demux/1
  Demux/3 -> psi_dot/1
  Demux/2 -> theta_dot/1
  Demux/1 -> phi_dot/1

== system B4_quadcopter_model_discrete/Discrete Model - Inner Loop Only/Discrete INDI Controller Cascaded/INTERNAL REFERENCE MODEL ATTITUDE/euler rates to body rates ==
  phi_dot : Inport
  theta_dot : Inport  Port=2
  psi_dot : Inport  Port=3
  Demux : Demux  Outputs=3
  Matrix Multiply : Product  Multiplication=Matrix(*)
  Mux : Mux  Inputs=3
  p : Outport
  q : Outport  Port=2
  r : Outport  Port=3
  wires:
  phi_dot/1 -> Mux/1
  theta_dot/1 -> Mux/2
  psi_dot/1 -> Mux/3
  [R_discr] -> Matrix Multiply/1
  Mux/1 -> Matrix Multiply/2
  Matrix Multiply/1 -> Demux/1
  Demux/3 -> r/1
  Demux/2 -> q/1
  Demux/1 -> p/1

== system B4_quadcopter_model_discrete/Discrete Model - Inner Loop Only/Discrete INDI Controller Cascaded w// Actuator Compensation Double/Butterworth Lowpass 2nd Order3/Switch Case Action Subsystem ==
  In1 : Inport
  Action Port : ActionPort
  Constant5 : Constant  Value=FILT_CUTOFF  SampleTime=sampling_time
  Lowpass2 : cstblocks/Linear Parameter Varying/Discrete Varying Lowpass  N=2  w0=0  Ts=sampling_time
      settings: SourceProductBaseCode=CT
  Out1 : Outport
  wires:
  Constant5/1 -> Lowpass2/2
  In1/1 -> Lowpass2/1
  Lowpass2/1 -> Out1/1

== system B4_quadcopter_model_discrete/Discrete Model - Inner Loop Only/Discrete INDI Controller Cascaded w// Actuator Compensation Double/Butterworth Lowpass 2nd Order3/Switch Case Action Subsystem1 ==
  In1 : Inport
  Action Port : ActionPort
  Out1 : Outport
  wires:
  In1/1 -> Out1/1

== system B4_quadcopter_model_discrete/Discrete Model - Inner Loop Only/Discrete INDI Controller Cascaded w// Actuator Compensation Double/INTERNAL REFERENCE MODEL ATTITUDE/body rates to euler rates ==
  p : Inport
  q : Inport  Port=2
  r : Inport  Port=3
  Demux : Demux  Outputs=3
  Matrix Multiply : Product  Multiplication=Matrix(*)
  Mux : Mux  Inputs=3
  phi_dot : Outport
  theta_dot : Outport  Port=2
  psi_dot : Outport  Port=3
  wires:
  p/1 -> Mux/1
  q/1 -> Mux/2
  r/1 -> Mux/3
  [T_discr] -> Matrix Multiply/1
  Mux/1 -> Matrix Multiply/2
  Matrix Multiply/1 -> Demux/1
  Demux/3 -> psi_dot/1
  Demux/2 -> theta_dot/1
  Demux/1 -> phi_dot/1

== system B4_quadcopter_model_discrete/Discrete Model - Inner Loop Only/Discrete INDI Controller Cascaded w// Actuator Compensation Double/INTERNAL REFERENCE MODEL ATTITUDE/euler rates to body rates ==
  phi_dot : Inport
  theta_dot : Inport  Port=2
  psi_dot : Inport  Port=3
  Demux : Demux  Outputs=3
  Matrix Multiply : Product  Multiplication=Matrix(*)
  Mux : Mux  Inputs=3
  p : Outport
  q : Outport  Port=2
  r : Outport  Port=3
  wires:
  phi_dot/1 -> Mux/1
  theta_dot/1 -> Mux/2
  psi_dot/1 -> Mux/3
  [R_discr] -> Matrix Multiply/1
  Mux/1 -> Matrix Multiply/2
  Matrix Multiply/1 -> Demux/1
  Demux/3 -> r/1
  Demux/2 -> q/1
  Demux/1 -> p/1

== system B4_quadcopter_model_discrete/Discrete Model - Inner Loop Only/Discrete INDI Controller Cascaded w// Actuator Compensation Double/Pitch Jerk Compensation/Butterworth Lowpass 2nd Order2 ==
  state estimate : Inport
  Constant5 : Constant  Value=FILT_CUTOFF  SampleTime=sampling_time
  Lowpass2 : cstblocks/Linear Parameter Varying/Discrete Varying Lowpass  N=2  w0=0  Ts=sampling_time
      settings: SourceProductBaseCode=CT
  Out : Outport
  wires:
  Constant5/1 -> Lowpass2/2
  Lowpass2/1 -> Out/1
  state estimate/1 -> Lowpass2/1

== system B4_quadcopter_model_discrete/Discrete Model - Inner Loop Only/Discrete INDI Controller Cascaded w// Actuator Compensation Double/Pitch Jerk Compensation/Model Based State Estimate ==
  Mux : Mux  Inputs=12
  state estimate : Outport
  wires:
  [Az] -> Mux/9
  [Vy] -> Mux/2
  [q] -> Mux/11
  [phi] -> Mux/4
  [Ay] -> Mux/8
  [p] -> Mux/10
  [psi] -> Mux/6
  [Ax] -> Mux/7
  [r] -> Mux/12
  [Vx] -> Mux/1
  [theta] -> Mux/5
  [Vz] -> Mux/3
  Mux/1 -> state estimate/1  "plant based"

== system B4_quadcopter_model_discrete/Discrete Model - Inner Loop Only/Discrete INDI Controller Cascaded w// Actuator Compensation Double/Pitch Jerk Compensation/State Filtered ==
  Mux : Mux  Inputs=12
  state filtered : Outport
  wires:
  [Az_f] -> Mux/9
  [Vy_f] -> Mux/2
  [q_f] -> Mux/11
  [phi_f] -> Mux/4
  [Ay_f] -> Mux/8
  [p_f] -> Mux/10
  [psi_f] -> Mux/6
  [Ax_f] -> Mux/7
  [r_f] -> Mux/12
  [Vx_f] -> Mux/1
  [theta_f] -> Mux/5
  [Vz_f] -> Mux/3
  Mux/1 -> state filtered/1  "plant based"
